simulink library "SUS_IOP_WD"  (Simulink 7.5)
settings: Solver=ode45  StartTime=0.0  StopTime=10.0  RelTol=1e-3
libraries: OSEM_WD x6
settings Model: Creator=controls  LastModifiedBy=controls

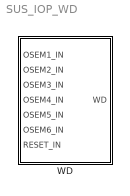
== system SUS_IOP_WD ==
  WD : Subsystem

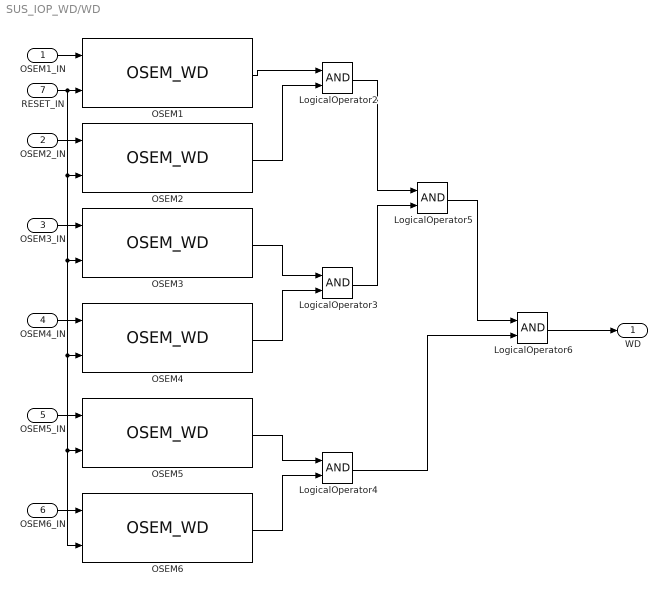
== system SUS_IOP_WD/WD ==
  OSEM1_IN : Inport
  OSEM2_IN : Inport  Port=2
  OSEM3_IN : Inport  Port=3
  OSEM4_IN : Inport  Port=4
  OSEM5_IN : Inport  Port=5
  OSEM6_IN : Inport  Port=6
  RESET_IN : Inport  Port=7
  LogicalOperator{2..6} (5 alike) : Logic  AllPortsSameDT=off  OutDataTypeMode=boolean  OutDataTypeStr=boolean
  OSEM{1..6} (6 alike) : OSEM_WD/OSEM_WD  SystemSampleTime=-1
  WD : Outport  OutDataType=fixdt(1, 16)  OutScaling=2^0
  wires:
  OSEM1_IN/1 -> OSEM1/1
  OSEM2_IN/1 -> OSEM2/1
  OSEM3_IN/1 -> OSEM3/1
  OSEM4_IN/1 -> OSEM4/1
  OSEM5_IN/1 -> OSEM5/1
  OSEM6_IN/1 -> OSEM6/1
  OSEM1/1 -> LogicalOperator2/1
  OSEM2/1 -> LogicalOperator2/2
  OSEM3/1 -> LogicalOperator3/1
  OSEM4/1 -> LogicalOperator3/2
  OSEM5/1 -> LogicalOperator4/1
  OSEM6/1 -> LogicalOperator4/2
  LogicalOperator2/1 -> LogicalOperator5/1
  LogicalOperator3/1 -> LogicalOperator5/2
  LogicalOperator5/1 -> LogicalOperator6/1
  LogicalOperator4/1 -> LogicalOperator6/2
  LogicalOperator6/1 -> WD/1
  RESET_IN/1 -> OSEM1/2, OSEM2/2, OSEM3/2, OSEM4/2, OSEM5/2, OSEM6/2
